simulink model "sitlFromRecordedData"  (R2024b)
settings: Solver=FixedStepAuto  StartTime=0.0  StopTime=10.0  FixedStep=1/simset.simHz  RelTol=1e-3
undefined symbols (not defined in the file): createArray, imuHz, simset
libraries: ros2lib x4
settings Model: PacingRate=10  Creator=Alyssa  LastModifiedBy=Alyssa

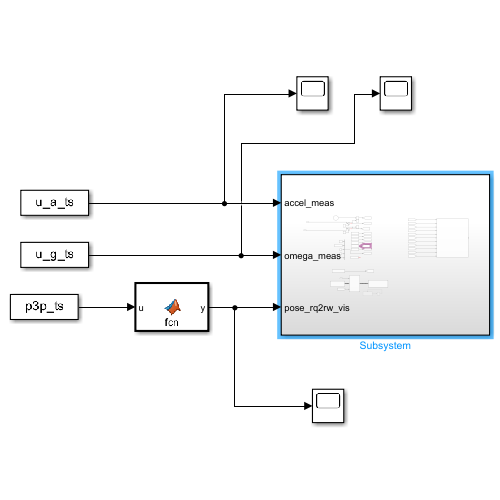
[thumbnail: Simulink's stored preview of the top-level diagram]
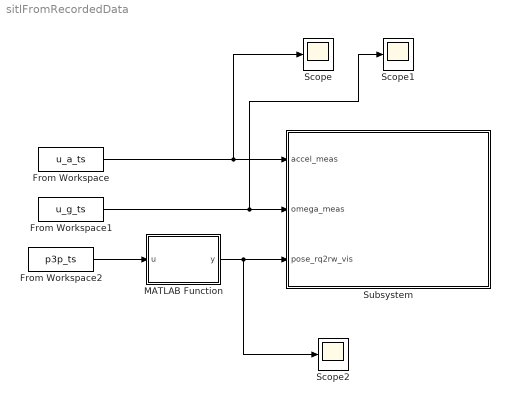
== system sitlFromRecordedData ==
  From Workspace : FromWorkspace  VariableName=u_a_ts  SampleTime=1/simset.simHz  Interpolate=off  OutputAfterFinalValue=Holding final value
  From Workspace1 : FromWorkspace  VariableName=u_g_ts  SampleTime=1/simset.simHz  Interpolate=off  OutputAfterFinalValue=Holding final value
  From Workspace2 : FromWorkspace  VariableName=p3p_ts  SampleTime=1/simset.simHz  Interpolate=off  OutputAfterFinalValue=Holding final value
  MATLAB Function : MATLAB Function  TreatAsAtomicUnit=on
  Scope : Scope
  Scope1 : Scope
  Scope2 : Scope
  Subsystem : Subsystem
  wires:
  From Workspace2/1 -> MATLAB Function/1(u)
  From Workspace1/1 -> Scope1/1, Subsystem/2(omega_meas)
  From Workspace/1 -> Scope/1, Subsystem/1(accel_meas)
  MATLAB Function/1(y) -> Scope2/1, Subsystem/3(pose_rq2rw_vis)

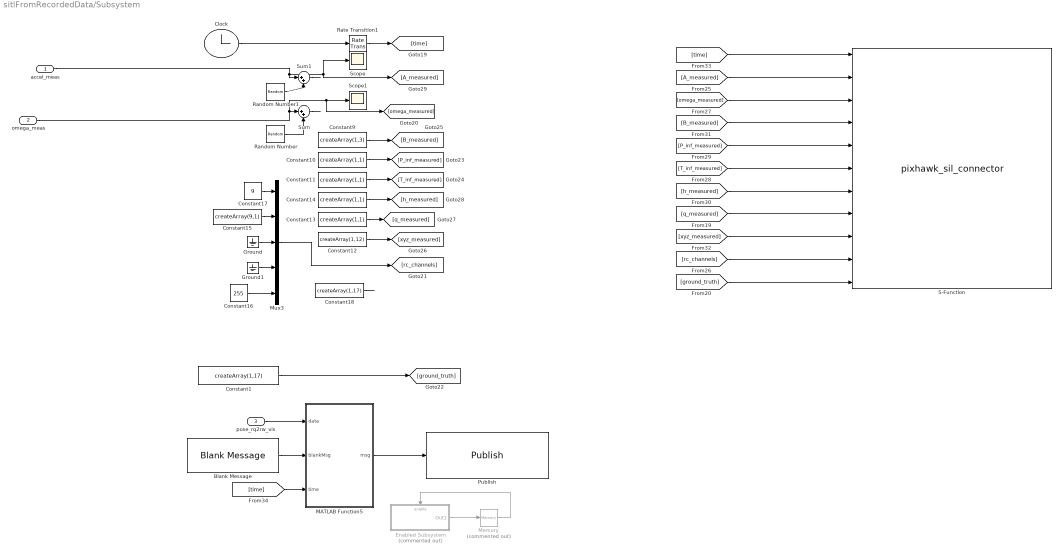
== system sitlFromRecordedData/Subsystem ==
  accel_meas : Inport
  omega_meas : Inport  Port=2
  pose_rq2rw_vis : Inport  Port=3
  Blank Message : ros2lib/Blank Message  messageClass=Message  entityType=px4_msgs/VehicleOdometry  messageType=px4_msgs/VehicleOdometry  SampleTime=1/simset.fps
  Clock : Clock
  Constant1 : Constant  Value=createArray(1,17)
  Constant{10..11,13..14} (4 alike) : Constant  Value=createArray(1,1)
  Constant12 : Constant  Value=createArray(1,12)
  Constant15 : Constant  Value=createArray(9,1)
  Constant16 : Constant  Value=255
  Constant17 : Constant  Value=9
  Constant18 : Constant  Value=createArray(1,17)
  Constant9 : Constant  Value=createArray(1,3)
  Enabled Subsystem : Subsystem  Commented=on  TreatAsAtomicUnit=on
  Ground : Ground
  Ground1 : Ground
  MATLAB Function5 : MATLAB Function  TreatAsAtomicUnit=on
  Memory : Memory  Commented=on  InitialCondition=1
  Mux3 : Mux  Inputs=5
  Publish : ros2lib/Publish  topicSource=Specify your own  topic=/fmu/in/vehicle_visual_odometry  messageType=px4_msgs/VehicleOdometry  QOSHistory=Keep last  QOSDepth=1  QOSReliability=Reliable  QOSDurability=Volatile  QOSDeadline=Inf  QOSLifespan=Inf  QOSLiveliness=Automatic  QOSLeaseDuration=Inf  QOSAvoidROSNamespaceConventions=off
  Random Number : RandomNumber  Mean=[0 0 0]  Variance=[0.01 0.01 0.01]*0.01  SampleTime=1/imuHz
  Random Number1 : RandomNumber  Mean=[0 0 0]  Variance=[0.1 0.1 0.1]*0.01  SampleTime=1/imuHz
  Rate Transition1 : RateTransition  OutPortSampleTime=0.004
  S-Function : S-Function  FunctionName=pixhawk_sil_connector  SFunctionDeploymentMode=off  EnableBusSupport=off
  Scope : Scope
  Scope1 : Scope
  Sum : Sum  Inputs=|++
  Sum1 : Sum  Inputs=|++
  wires:
  Ground/1 -> Mux3/3
  Constant14/1 -> [h_measured]
  pose_rq2rw_vis/1 -> MATLAB Function5/1(data)
  accel_meas/1 -> Sum1/1, [A_measured], Scope/1
  [T_inf_measured] -> S-Function/6
  Constant17/1 -> Mux3/1
  Blank Message/1 -> MATLAB Function5/2(blankMsg)
  [ground_truth] -> S-Function/11
  [omega_measured] -> S-Function/3
  [time] -> MATLAB Function5/3(time)
  Constant13/1 -> [q_measured]
  [rc_channels] -> S-Function/10
  [A_measured] -> S-Function/2
  Rate Transition1/1 -> [time]
  Memory/1 -> Enabled Subsystem/Enable
  [h_measured] -> S-Function/7
  Constant11/1 -> [T_inf_measured]
  Constant1/1 -> [ground_truth]
  Clock/1 -> Rate Transition1/1
  [time] -> S-Function/1
  Sum1/1 -> ?
  Ground1/1 -> Mux3/4
  omega_meas/1 -> Sum/1, Scope1/1, [omega_measured]
  Random Number1/1 -> Sum1/2
  Random Number/1 -> Sum/2
  Sum/1 -> ?
  Constant15/1 -> Mux3/2
  Constant16/1 -> Mux3/5
  Enabled Subsystem/1(Out1) -> Memory/1
  [xyz_measured] -> S-Function/9
  [q_measured] -> S-Function/8
  Constant12/1 -> [xyz_measured]
  [P_inf_measured] -> S-Function/5
  Mux3/1 -> [rc_channels]
  Constant9/1 -> [B_measured]
  Constant10/1 -> [P_inf_measured]
  MATLAB Function5/1(msg) -> Publish/1
  [B_measured] -> S-Function/4
  Constant18/1 -> ?

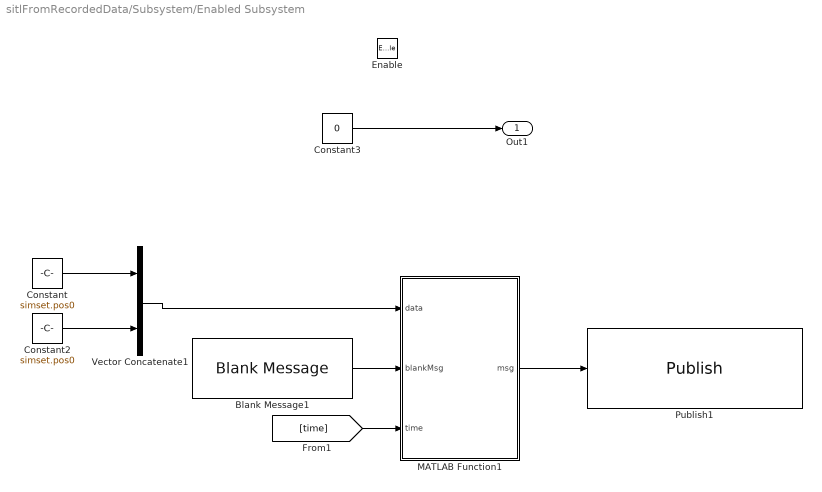
== system sitlFromRecordedData/Subsystem/Enabled Subsystem ==
  Enable : EnablePort
  Blank Message1 : ros2lib/Blank Message  messageClass=Message  entityType=px4_msgs/VehicleOdometry  messageType=px4_msgs/VehicleOdometry  SampleTime=inf
  Constant : Constant  Value=simset.pos0
  Constant2 : Constant  Value=simset.pos0
  Constant3 : Constant  Value=0
  MATLAB Function1 : MATLAB Function  TreatAsAtomicUnit=on
  Publish1 : ros2lib/Publish  topicSource=Specify your own  topic=/fmu/in/vehicle_visual_odometry  messageType=px4_msgs/VehicleOdometry  QOSHistory=Keep last  QOSDepth=1  QOSReliability=Reliable  QOSDurability=Volatile  QOSDeadline=Inf  QOSLifespan=Inf  QOSLiveliness=Automatic  QOSLeaseDuration=Inf  QOSAvoidROSNamespaceConventions=off
  Vector Concatenate1 : Concatenate
  Out1 : Outport
  wires:
  Constant3/1 -> Out1/1
  Constant/1 -> Vector Concatenate1/1
  Blank Message1/1 -> MATLAB Function1/2(blankMsg)
  Constant2/1 -> Vector Concatenate1/2
  [time] -> MATLAB Function1/3(time)
  MATLAB Function1/1(msg) -> Publish1/1
  Vector Concatenate1/1 -> MATLAB Function1/1(data)

== matlab function sitlFromRecordedData/MATLAB Function ==
  data: u input; y output
function y = fcn(u)


if vecnorm(u,2,2) ==0
    y = nan(7,1);
else
    y = u;
end

== matlab function sitlFromRecordedData/Subsystem/Enabled Subsystem/MATLAB Function1 ==
  settings: updateMethod=DISCRETE  sampleTime=0.04
  data: data input; blankMsg input Bus: SL_Bus_px4_msgs_VehicleOdometry; msg output Bus: SL_Bus_px4_msgs_VehicleOdometry; time input
function msg = fcn(data, blankMsg, time)

%msg = ros2message("px4_msgs/VehicleOdometry");
msg = blankMsg;

%populate headers and other overhead info
timestamp_us = time * 1e6;
msg.timestamp = timestamp_us;
msg.timestamp_sample = timestamp_us;

msg.pose_frame = uint8(1); %set to POSE_FRAME_NED

msg.reset_counter = uint8(0);
msg.quality = int8(1);

%populate pose
%quat = tform2quat(data)';
%pos = tform2trvec(data)';
eul = data(4:6);
quat =eul2quat(eul', 'XYZ')';
pos = data(1:3);

msg.position = single(pos);
msg.q = [single(quat(1)); single(quat(2)); single(quat(3)); single(quat(4))];

% %populate covariance - if all zeroes, px4 will reject
msg.position_variance = single([0.01; 0.01; 0.01]);
msg.orientation_variance = single([0.01; 0.01; 0.01]);

%disp('Sent pose');

== matlab function sitlFromRecordedData/Subsystem/MATLAB Function5 ==
  settings: updateMethod=DISCRETE  sampleTime=0.04
  data: data input; blankMsg input Bus: SL_Bus_px4_msgs_VehicleOdometry; msg output Bus: SL_Bus_px4_msgs_VehicleOdometry; time input
function msg = fcn(data, blankMsg, time)

%msg = ros2message("px4_msgs/VehicleOdometry");
msg = blankMsg;

%populate headers and other overhead info
timestamp_us = time * 1e6;
msg.timestamp = timestamp_us;
msg.timestamp_sample = timestamp_us;

msg.pose_frame = uint8(1); %set to POSE_FRAME_NED

msg.reset_counter = uint8(0);
msg.quality = int8(1);

%populate pose
%quat = tform2quat(data)';
%pos = tform2trvec(data)';
quat = data(4:7);
pos = data(1:3);

msg.position = single(pos);
msg.q = [single(quat(1)); single(quat(2)); single(quat(3)); single(quat(4))];

% %populate covariance - if all zeroes, px4 will reject
%msg.position_variance = single([0.2; 0.2; 0.2]); %(m^2)
%msg.orientation_variance = single([0.1; 0.1; 0.1]); %(rad^2)

msg.position_variance = single([0.13^2; 0.13^2; 0.13^2]); %(m^2)
msg.orientation_variance = single([0.1; 0.1; 0.1]); %(rad^2)


%disp('Sent pose');
